simulink model "Case_1"  (R2023b)
settings: Solver=VariableStepAuto  StartTime=0.0  StopTime=1  FixedStep=Ts  RelTol=1e-3  EnableMultiTasking=on
PreLoadFcn:
  | %% Parameters for BLDC Speed Control Example
  | 
  | % This example shows how to control the rotor speed in a BLDC based
  | % electrical drive. An ideal torque source provides the load. The Control
  | % subsystem uses a PI-based cascade control structure with an outer speed
  | % control loop and an inner dc-link voltage control loop. The dc-link
  | % voltage is adjusted through a DC-DC buck converter. The BLDC is fed by
  | % a controlled three-phase inverter. The gate signals for the inverter
  | % are obtained from hall signals. The simulation uses speed steps. The
  | % Scopes subsystem contains scopes that allow you to see the simulation
  | % results.
  | 
  | % Copyright 2017 The MathWorks, Inc.
  | 
  | %% Machine Parameters
  | p    = 4;        % Number of pole pairs
  | Rs   = 0.1;      % Stator resistance per phase           [Ohm]
  | Ls   = 1e-4;     % Stator self-inductance per phase, Ls  [H]
  | Ms   = 1e-5;     % Stator mutual inductance, Ms          [H]
  | psim = 0.0175;   % Maximum permanent magnet flux linkage [Wb]
  | Jm   = 0.0005;   % Rotor inertia                         [Kg*m^2]
  | 
  | %% Control Parameters
  | Ts  = 5e-6;  % Fundamental sample time            [s]
  | Tsc = 1e-4;  % Sample time for inner control loop [s]
  | Vdc = 48;    % Maximum DC link voltage            [V]
  | Kpw = 0.1;   % Proportional gain speed controller
  | Kiw = 15;    % Integrator gain speed controller
  | Kpv = 0.1;   % Proportional gain voltage controller
  | Kiv = 0.5;   % Integrator gain voltage controller
libraries: nesl_utility x16, fl_lib x13, ee_lib x6, slctrl_autotuning x2, eeDiscretePi x2, eeGeneralControl x1, eePwmGenerator x1, spsTriangleGeneratorLib x1
CloseFcn:
  | try,close(h1_pe_bldc_speed_control),end
  | clear h1_pe_bldc_speed_control
  | 
  | clear simlog_pe_bldc_speed_control
  | clear logsout_pe_bldc_speed_control
Description:
  | BLDC Speed Control
settings Model: Creator=The MathWorks, Inc.  LastModifiedBy=HP
settings SolverCC: AllowMultiTaskInputOutput=on  AlgebraicLoopSolver=TrustRegion  AutoInsertRateTranBlk=on  MinimalZcImpactIntegration=on  MaxZcPerStep=1
settings DataIOCC: MaxDataPoints=210000  SaveOutput=off  SignalLogging=off  DSMLogging=off  SaveTime=off  SignalLoggingName=logsout_pe_bldc_speed_control
settings OptimizationCC: ReuseModelBlockBuffer=off  LifeSpan=inf
settings DebuggingCC: UnderspecifiedInitializationDetection=Classic  MergeDetectMultiDrivingBlocksExec=none  UnconnectedInputMsg=warning  UnconnectedOutputMsg=warning  UnconnectedLineMsg=warning  PregeneratedLibrarySubsystemCodeDiagnostic=none  SFUnexpectedBacktrackingDiag=warning  SFNoUnconditionalDefaultTransitionDiag=warning  SFExecutionAtInitializationDiag=none  ArithmeticOperatorsInVariantConditions=warning
settings ModelReferenceCC: EnableRefExpFcnMdlSchedulingChecks=on
settings SFSimCC: SimUseLocalCustomCode=off  CustomCodeUndefinedFunction=UseInterfaceOnly
settings RTWCC: RTWUseLocalCustomCode=off  CheckMdlBeforeBuild=Warning  DLArmComputeVersion=19.05
settings CodeAppCC: StateflowObjectComments=on
settings ConfigComp: CovMetricSettings=dw  CovSaveCumulativeToWorkspaceVar=on  CovSaveSingleToWorkspaceVar=on  CovExternalEMLEnable=off
settings SimscapeCC: SimscapeNormalizeSystem=off  SimscapeLogSimulationStatistics=on  SimscapeLogName=simlog_pe_bldc_speed_control  SimscapeLogDataHistory=210000

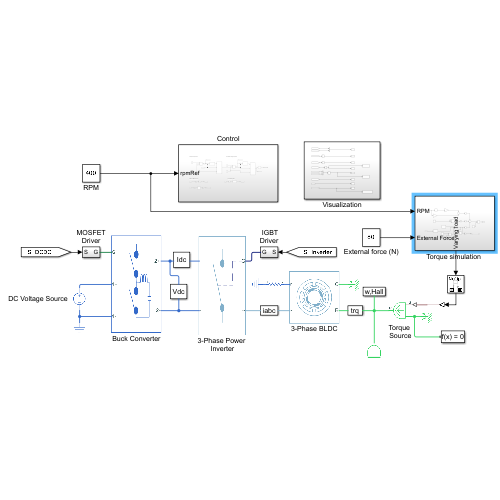
[thumbnail: Simulink's stored preview of the top-level diagram]
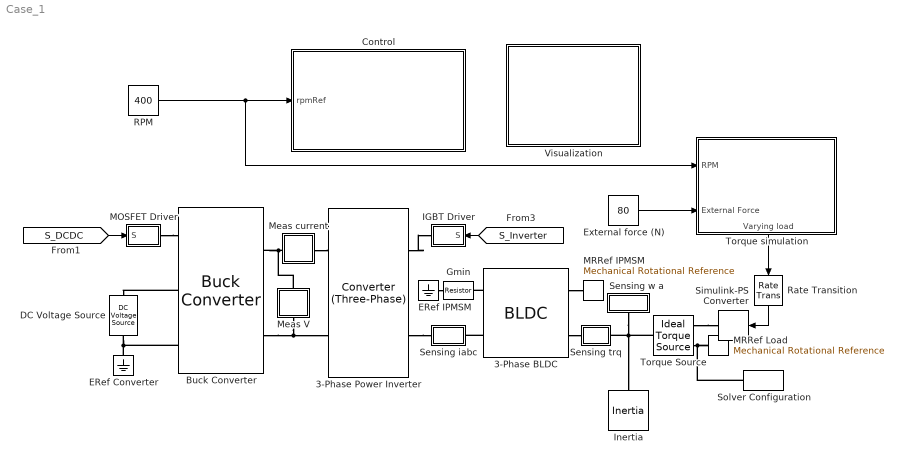
== system Case_1 ==
  " DC Voltage Source" : fl_lib/Electrical/Electrical Sources/DC Voltage Source  v0=Vdc V
  " IGBT Driver" : Subsystem
  3-Phase BLDC : ee_lib/Electromechanical/Permanent Magnet/BLDC  port_option=ee.enum.threePhasePort.composite  rotor_param=1  pm_flux_linkage=psim Wb  theta_constant=pi / (2*p) rad  emf_max=9.6 V  w_meas=600 rpm  DphiDtheta_tab=[0, -.1528, -.1528, .1528, .1528, 0] Wb/rad  back_emf_tab=[0, -9.6, -9.6, 9.6, 9.6, 0] V  rotor_angle_tab=[0, 7.5, 22.5, 37.5, 52.5, 60] deg  nPolePairs=p  axes_param=1  winding_type=ee.enum.statorconnection.wye  stator_param=2  machine_param=ee.enum.dqparameterization.constant  Ld=0.00022 H  Lq=0.00022 H  idVec=[-200, 0, 200] A  iqVec=[-200, 0, 200] A  LdMatrix=0.00022 * ones(3, 3) H  LqMatrix=0.00022 * ones(3, 3) H  L0=0.00016 H  Ls=Ls H  Lm=0 H  Ms=Ms H  Rs=Rs Ohm  zero_sequence=ee.enum.park.zerosequence.include  loss_param=ee.enum.ironloss.none  losses_oc=[0, 0, 0] W  losses_sc=[0, 0, 0] W  f_losses=60 Hz  Isc_losses=95 A  J=0.01 kg*m^2  lam=0 N*m/(rad/s)  i_d_specify=off  i_d_priority=None  i_d=0 A  i_d_nominal_specify=off  i_d_nominal_unit=A  i_d_nominal_value=1  i_q_specify=off  i_q_priority=None  i_q=0 A  i_q_nominal_specify=off  i_q_nominal_unit=A  i_q_nominal_value=1  torque_specify=off  torque_priority=None  torque=0 N*m  torque_nominal_specify=off  torque_nominal_unit=N*m  torque_nominal_value=1  angular_velocity_specify=off  angular_velocity_priority=High  angular_velocity=0 rpm  angular_velocity_nominal_specify=off  angular_velocity_nominal_unit=rpm  angular_velocity_nominal_value=1  angular_position_specify=off  angular_position_priority=High  angular_position=0 deg  angular_position_nominal_specify=off  angular_position_nominal_unit=deg  angular_position_nominal_value=1  alpha=3.93e-3 1/K  alpha_flux=-0.001 1/K  Tmeas=298.15 K  stator_thermal_mass=100 J/K  rotor_thermal_mass=200 J/K  Rm_percent_rotor=90  Rd_percent_rotor=30  temperatureA_specify=off  temperatureA_priority=High  temperatureA=25 degC  temperatureA_nominal_specify=off  temperatureA_nominal_unit=degC  temperatureA_nominal_value=1  temperatureB_specify=off  temperatureB_priority=High  temperatureB=25 degC  temperatureB_nominal_specify=off  temperatureB_nominal_unit=degC  temperatureB_nominal_value=1  temperatureC_specify=off  temperatureC_priority=High  temperatureC=25 degC  temperatureC_nominal_specify=off  temperatureC_nominal_unit=degC  temperatureC_nominal_value=1  temperatureR_specify=off  temperatureR_priority=High  temperatureR=25 degC  temperatureR_nominal_specify=off  temperatureR_nominal_unit=degC  temperatureR_nominal_value=1
      settings: InternalSimscapePortConfiguration="{\"Bottom\":[],\"Left\":[{\"id\":\"N\",\"label\":\"~\",\"type\":\"foundation.electrical.three_phase\"},{\"id\":\"n\",\"label\":\"n\",\"type\":\"foundation.electrical.electrical\"}],\"Right\":[{\"id\":\"R\",\"label\":\"R\",\"type\":\"foundation.mechanical.rotational.rotational\"},{\"id\":\"C\",\"label\":\"C\",\"type\":\"foundation.mechanical.rotational.rotational\"}],\"Top\":[]}"
  3-Phase Power Inverter : ee_lib/Semiconductors & Converters/Converters/Converter (Three-Phase)  port_option=ee.enum.threePhasePort.composite  device_type=3  K=0  Vf=0.8 V  Ron=0.001 Ohm  Rds=0.001 Ohm  Goff=1e-5 1/Ohm  Vgt=1 V  Vgt_off=-1 V  Ih=1 A  Vth=0.5 V  diode_param=2  diode_Vf=0.8 V  diode_Ron=0.001 Ohm  diode_Goff=1e-5 1/Ohm  diode_C=50 nF  diode_iRM=-235 A  diode_iF=300 A  diode_idot=-50 A/us  diode_trr_param=1  diode_trr_factor=3  diode_trr=15 us  diode_Qrr=1.5e+3 s*uA  snubber_type=0  Cs=1e-7 F  Rs=0.1 Ohm
  Buck Converter : ee_lib/Semiconductors & Converters/Converters/Buck Converter  port_option=ee.enum.controlport.ps  device_type=4  Vf=0.8 V  Ron=0.001 Ohm  Rds=0.001 Ohm  Goff=1e-5 1/Ohm  Vgt=1 V  Vgt_off=-1 V  Ih=1 A  Vth=0.5 V  K=0  diode_param=2  diode_Vf=0.8 V  diode_Ron=0.001 Ohm  diode_Goff=1e-5 1/Ohm  diode_C=50 nF  diode_iRM=-235 A  diode_iF=300 A  diode_idot=-50 A/us  diode_trr_param=1  diode_trr_factor=3  diode_trr=15 us  diode_Qrr=1500 s*uA  Lf=220 uH  Rl=0 Ohm  Cf=10 uF  Rf=.25 Ohm  snubber_type=1  Cs=1e-7 F  Rs=0.1 Ohm  iL_specify=off  iL_priority=High  iL=0 A  iL_nominal_specify=off  iL_nominal_unit=A  iL_nominal_value=1  vc_specify=off  vc_priority=High  vc=0 V  vc_nominal_specify=off  vc_nominal_unit=V  vc_nominal_value=1
      settings: InternalSimscapePortConfiguration="{\"Bottom\":[],\"Left\":[{\"id\":\"G\",\"label\":\"G\",\"type\":\"foundation.electrical.four_phase\"},{\"id\":\"p1\",\"label\":\"1+\",\"type\":\"foundation.electrical.electrical\"},{\"id\":\"n1\",\"label\":\"1-\",\"type\":\"foundation.electrical.electrical\"}],\"Right\":[{\"id\":\"p2\",\"label\":\"2+\",\"type\":\"foundation.electrical.electrical\"},{\"id\":\"n2\",\"label\":\"2-\",\"type\":\"foundation.electrical.electrical\"}],\"Top\":[]}"
  Control : Subsystem
  ERef Converter : fl_lib/Electrical/Electrical Elements/Electrical Reference
  ERef IPMSM : fl_lib/Electrical/Electrical Elements/Electrical Reference
  External force (N) : Constant  Value=80
  Gmin : fl_lib/Electrical/Electrical Elements/Resistor  R=1e9 Ohm  i_specify=off  i_priority=High  i=0 A  i_nominal_specify=off  i_nominal_unit=A  i_nominal_value=1  v_specify=off  v_priority=High  v=0 V  v_nominal_specify=off  v_nominal_unit=V  v_nominal_value=1
  Inertia : fl_lib/Mechanical/Rotational Elements/Inertia  inertia=Jm kg*m^2  num_ports=foundation.enum.numPorts2.one  w_specify=on  w_priority=High  w=0 rpm  w_nominal_specify=off  w_nominal_unit=rad/s  w_nominal_value=1  t_specify=off  t_priority=High  t=0 N*m  t_nominal_specify=off  t_nominal_unit=N*m  t_nominal_value=1
  "MOSFET Driver " : Subsystem
  MRRef IPMSM : fl_lib/Mechanical/Rotational Elements/Mechanical Rotational Reference
  MRRef Load : fl_lib/Mechanical/Rotational Elements/Mechanical Rotational Reference
  Meas V : Subsystem
      mask Display: disp('Vdc')
  Meas current : Subsystem
      settings: PortSchema="{\"entries\":[{\"content\":{\"sides\":[{\"content\":{},\"type\":\"ConnectorPlacement.EquallySpacedRectSide\",\"uuid\":\"82ca6d8b-4f1d-482c-9132-345f1111dd8f\"},{\"content\":{\"side\":\"RIGHT\"},\"type\":\"ConnectorPlacement.EquallySpacedRectSide\",\"uuid\":\"46eb7c2e-5f99-46a8-b5a6-ad4c053dfe5d\"},{\"content\":{\"connectorIds\":[\"LConn1\"],\"side\":\"TOP\"},\"type\":\"ConnectorPlacement.EquallySpacedRectSide\",\"uuid\":\"5837dc94-a870-4fd0-9d92-a25376552da6\"},{\"content\":{\"connectorIds\":[\"RConn1\"],\"side\":\"BOTTOM\"},\"type\":\"ConnectorPlacement.EquallySpacedRectSide\",\"uuid\":\"ef4e5c2a-3af4-4835-9bd1-a57a6b683b63\"}]},\"type\":\"ConnectorPlacement.EquallySpacedConnector\",\"uuid\":\"b19ad980-4c6f-4f24-94cb-fca13afdc426\"}],\"packageUris\":[\"http://schema.mathworks.com/mf0/Connector/R2020b\"],\"version\":\"1.0\"}"
      mask Display: disp('Idc')
  RPM : Constant  Value=400
  Rate Transition : RateTransition  OutPortSampleTimeOpt=Inherit
  Sensing trq : Subsystem
      mask Display: disp('trq')
  Sensing w a : Subsystem
      mask Display: disp('w,Hall')
  Sensing iabc : Subsystem
      mask Display: disp('iabc')
  Simulink-PS Converter : nesl_utility/Simulink-PS Converter  PhysicalDomain=network_engine_domain  SubClassName=ps_input  LeftPortType=input  RightPortType=output  PseudoPeriodic=off  Frequencies=[]  NoiseDistribution=none  NoiseParameters=[]  Unit=N*m  AffineConversion=on  FilteringAndDerivatives=zero  SimscapeFilterOrder=1  InputFilterTimeConstant=0.001  UdotUserProvided=1
  Solver Configuration : nesl_utility/Solver Configuration  PhysicalDomain=network_engine_domain  SubClassName=solver  LeftPortType=input  RightPortType=generic  Tones=[]  Harmonics=[]  SimulateNoise=off  Profile=off  UseLocalSampling=off  EnableSwitchedLinearOptims=on  FrequencyDomain=off  UseCCode=off  RelTol=0.001  AbsTol=1e-06  MinStep=1e-09  ToWorkspace=off  RevertToSquareIcSolve=off  NumHomotopyIterations=100  PhasorMode=off  PhasorModeNumHarmonics=1  ConsistencySolver=NEWTON_FTOL  IndexReductionMethod=DerivativeReplacement  DoDC=off  ResidualTolerance=1e-9  ConsistencyTolSource=GLOBAL  ConsistencyAbsTol=0.001  ConsistencyRelTol=0.001  ConsistencyTolFactor=0.001  UseLocalSolver=on  LocalSolverChoice=NE_BACKWARD_EULER_ADVANCER  ResolveIndetEquations=on  FunctionEvalNumThread=1  LocalSolverSampleTime=Ts  DoFixedCost=on  MaxNonlinIter=4  MaxModeIter=2  ComputeImpulses=off  ImpulseIterations=2  LinearAlgebra=Sparse  LinearAlgebraNumThread=0  EquationFormulation=NE_TIME_EF  DelaysMemoryBudget=1024  AutomaticFiltering=on  FilteringTimeConstant=0.001  PartitionStorageMethod=AS_NEEDED  PartitionMemoryBudget=1024  PartitionMethod=FAST  MultibodyUseLocalSolver=off  MultibodyLocalSolverChoice=ODE1  MultibodyLocalSolverSampleTime=0.001
  Torque Source : fl_lib/Mechanical/Mechanical Sources/Ideal Torque Source
  "Torque simulation " : Subsystem
      settings: PortSchema="{\"entries\":[{\"content\":{\"sides\":[{\"content\":{\"connectorIds\":[\"In1\",\"In2\"]},\"type\":\"ConnectorPlacement.EquallySpacedRectSide\",\"uuid\":\"4de94c05-994b-4a6b-aa57-8a8325026801\"},{\"content\":{\"side\":\"RIGHT\"},\"type\":\"ConnectorPlacement.EquallySpacedRectSide\",\"uuid\":\"9aab4c8e-5a08-4361-b962-7ff1ea4c45cd\"},{\"content\":{\"side\":\"TOP\"},\"type\":\"ConnectorPlacement.EquallySpacedRectSide\",\"uuid\":\"3907e8e7-ade8-4b6d-b9e3-a2c225338252\"},{\"content\":{\"connectorIds\":[\"Out1\"],\"side\":\"BOTTOM\"},\"type\":\"ConnectorPlacement.EquallySpacedRectSide\",\"uuid\":\"9adc3eea-f106-4f90-8d03-70cb44881ebc\"}]},\"type\":\"ConnectorPlacement.EquallySpacedConnector\",\"uuid\":\"d6098bb0-da6b-4857-a7db-fd24669e7041\"}],\"packageUris\":[\"http://schema.mathworks.com/mf0/Connector/R2020b\"],\"version\":\"1.0\"}"
  Visualization : Subsystem
  wires:
  [S_DCDC] -> "MOSFET Driver "/1(S)
  [S_Inverter] -> " IGBT Driver"/1(S)
  "Torque simulation "/1(Varying load) -> Rate Transition/1
  External force (N)/1 -> "Torque simulation "/2(External Force)
  RPM/1 -> "Torque simulation "/1(RPM), Control/1(rpmRef)
  Rate Transition/1 -> Simulink-PS Converter/1
  connections:
  Torque Source/LConn1 -- Sensing w a/LConn1 -- Sensing trq/RConn1 -- Inertia/LConn1
  ERef IPMSM/LConn1 -- Gmin/LConn1
  3-Phase BLDC/LConn2 -- Gmin/RConn1
  Torque Source/RConn1 -- Simulink-PS Converter/RConn1
  Torque Source/RConn2 -- Solver Configuration/RConn1 -- MRRef Load/LConn1
  3-Phase BLDC/LConn1 -- Sensing iabc/RConn1
  3-Phase BLDC/RConn2 -- MRRef IPMSM/LConn1
  3-Phase BLDC/RConn1 -- Sensing trq/LConn1
  Buck Converter/LConn2 -- " DC Voltage Source"/LConn1
  ERef Converter/LConn1 -- " DC Voltage Source"/RConn1 -- Buck Converter/LConn3
  "MOSFET Driver "/RConn1 -- Buck Converter/LConn1
  Buck Converter/RConn2 -- Meas V/RConn1 -- 3-Phase Power Inverter/RConn2
  Meas V/LConn1 -- Meas current/LConn1 -- Buck Converter/RConn1
  3-Phase Power Inverter/LConn1 -- " IGBT Driver"/RConn1
  3-Phase Power Inverter/LConn2 -- Sensing iabc/LConn1
  Meas current/RConn1 -- 3-Phase Power Inverter/RConn1

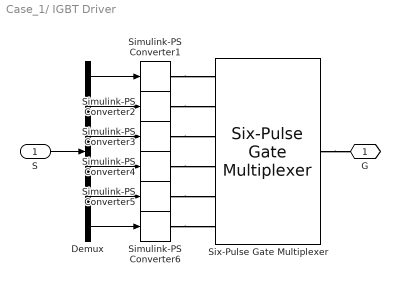
== system Case_1/ IGBT Driver ==
  S : Inport
  Demux : Demux  Outputs=6
  Simulink-PS Converter{1..6} (6 alike) : nesl_utility/Simulink-PS Converter  PhysicalDomain=network_engine_domain  SubClassName=ps_input  LeftPortType=input  RightPortType=output  PseudoPeriodic=off  Frequencies=[]  NoiseDistribution=none  NoiseParameters=[]  Unit=1  AffineConversion=off  FilteringAndDerivatives=zero  SimscapeFilterOrder=1  InputFilterTimeConstant=0.001  UdotUserProvided=1
  Six-Pulse Gate Multiplexer : ee_lib/Semiconductors & Converters/Converters/Six-Pulse Gate Multiplexer  port_option=ee.enum.controlport.ps
  G : PMIOPort  Side=Right
  wires:
  Demux/1 -> Simulink-PS Converter1/1
  S/1 -> Demux/1
  Demux/4 -> Simulink-PS Converter4/1
  Demux/2 -> Simulink-PS Converter2/1
  Demux/3 -> Simulink-PS Converter3/1
  Demux/5 -> Simulink-PS Converter5/1
  Demux/6 -> Simulink-PS Converter6/1
  connections:
  Six-Pulse Gate Multiplexer/RConn1 -- G/RConn1
  Simulink-PS Converter1/RConn1 -- Six-Pulse Gate Multiplexer/LConn1
  Simulink-PS Converter3/RConn1 -- Six-Pulse Gate Multiplexer/LConn3
  Simulink-PS Converter5/RConn1 -- Six-Pulse Gate Multiplexer/LConn5
  Simulink-PS Converter6/RConn1 -- Six-Pulse Gate Multiplexer/LConn6
  Simulink-PS Converter4/RConn1 -- Six-Pulse Gate Multiplexer/LConn4
  Simulink-PS Converter2/RConn1 -- Six-Pulse Gate Multiplexer/LConn2

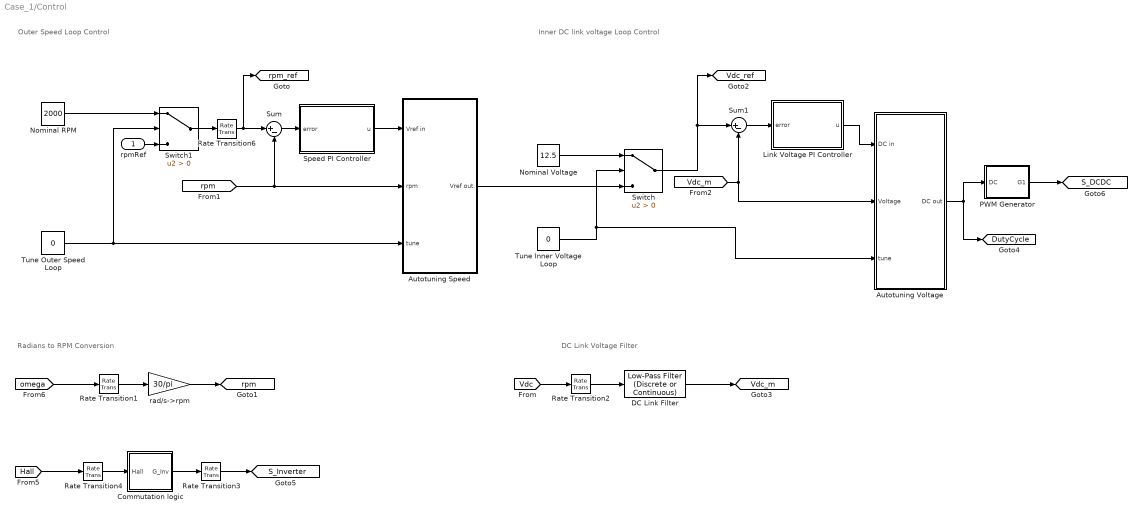
== system Case_1/Control ==
  note: Inner DC link voltage Loop Control
  note: Outer Speed Loop Control
  note: DC Link Voltage Filter
  note: Radians to RPM Conversion
  rpmRef : Inport
  Autotuning Speed : Subsystem
  Autotuning Voltage : Subsystem
  Commutation logic : Subsystem
  DC Link Filter : eeGeneralControl/Low-Pass Filter (Discrete or Continuous)  K=1  T=0.01  B=inf  A=-inf  init_option=Inherited from block input  x0=0  Ts=Tsc
  Link Voltage PI Controller : Subsystem
  Nominal RPM : Constant  Value=2000
  Nominal Voltage : Constant  Value=12.5
  PWM Generator : Subsystem
  Rate Transition1 : RateTransition
  Rate Transition2 : RateTransition
  Rate Transition3 : RateTransition  OutPortSampleTime=Ts
  Rate Transition4 : RateTransition  OutPortSampleTime=Tsc
  Rate Transition6 : RateTransition
  Speed PI Controller : Subsystem
  Sum : Sum  Inputs=|+-
  Sum1 : Sum  Inputs=|+-
  Switch : Switch  Criteria=u2 > Threshold  SaturateOnIntegerOverflow=off  InputSameDT=off
  Switch1 : Switch  Criteria=u2 > Threshold  SaturateOnIntegerOverflow=off  InputSameDT=off
  Tune Inner Voltage Loop : Constant  Value=0
  Tune Outer Speed Loop : Constant  Value=0
  rad/s->rpm : Gain  Gain=30/pi
  tag scope: DutyCycle=global, S_DCDC=global, S_Inverter=global, Vdc_m=global, Vdc_ref=global, rpm=global, rpm_ref=global
  wires:
  [omega] -> Rate Transition1/1
  [Hall] -> Rate Transition4/1
  rpmRef/1 -> Switch1/3
  Rate Transition6/1 -> [rpm_ref], Sum/1
  Rate Transition1/1 -> rad/s->rpm/1
  rad/s->rpm/1 -> [rpm]
  Rate Transition3/1 -> [S_Inverter]
  Rate Transition4/1 -> Commutation logic/1(Hall)
  Commutation logic/1(G_Inv) -> Rate Transition3/1
  PWM Generator/1(G1) -> [S_DCDC]
  [Vdc] -> Rate Transition2/1
  Autotuning Voltage/1(DC out) -> PWM Generator/1(DC), [DutyCycle]
  Rate Transition2/1 -> DC Link Filter/1
  DC Link Filter/1 -> [Vdc_m]
  Nominal Voltage/1 -> Switch/1
  Switch1/1 -> Rate Transition6/1
  Nominal RPM/1 -> Switch1/1
  Tune Inner Voltage Loop/1 -> Autotuning Voltage/3(tune), Switch/2
  Autotuning Speed/1(Vref out) -> Switch/3
  Tune Outer Speed Loop/1 -> Switch1/2, Autotuning Speed/3(tune)
  [rpm] -> Sum/2, Autotuning Speed/2(rpm)
  [Vdc_m] -> Sum1/2, Autotuning Voltage/2(Voltage)
  Sum/1 -> Speed PI Controller/1(error)
  Speed PI Controller/1(u) -> Autotuning Speed/1(Vref in)
  Link Voltage PI Controller/1(u) -> Autotuning Voltage/1(DC in)
  Sum1/1 -> Link Voltage PI Controller/1(error)
  Switch/1 -> Sum1/1, [Vdc_ref]

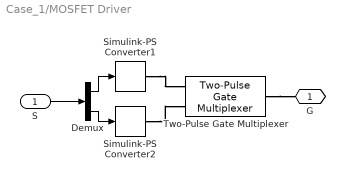
== system Case_1/MOSFET Driver  ==
  S : Inport
  Demux : Demux  Outputs=2
  Simulink-PS Converter1 : nesl_utility/Simulink-PS Converter  PhysicalDomain=network_engine_domain  SubClassName=ps_input  LeftPortType=input  RightPortType=output  PseudoPeriodic=off  Frequencies=[]  NoiseDistribution=none  NoiseParameters=[]  Unit=V  AffineConversion=off  FilteringAndDerivatives=zero  SimscapeFilterOrder=1  InputFilterTimeConstant=0.001  UdotUserProvided=1
  Simulink-PS Converter2 : nesl_utility/Simulink-PS Converter  PhysicalDomain=network_engine_domain  SubClassName=ps_input  LeftPortType=input  RightPortType=output  PseudoPeriodic=off  Frequencies=[]  NoiseDistribution=none  NoiseParameters=[]  Unit=V  AffineConversion=off  FilteringAndDerivatives=zero  SimscapeFilterOrder=1  InputFilterTimeConstant=0.001  UdotUserProvided=1
  Two-Pulse Gate Multiplexer : ee_lib/Semiconductors & Converters/Converters/Two-Pulse Gate Multiplexer  port_option=ee.enum.controlport.ps
      settings: InternalSimscapePortConfiguration="{\"Bottom\":[],\"Left\":[{\"id\":\"G1_ps\",\"label\":\"G1\",\"type\":\"input\"},{\"id\":\"G2_ps\",\"label\":\"G2\",\"type\":\"input\"}],\"Right\":[{\"id\":\"p\",\"label\":\"G\",\"type\":\"foundation.electrical.four_phase\"}],\"Top\":[]}"
  G : PMIOPort  Side=Right
  wires:
  Demux/1 -> Simulink-PS Converter1/1
  Demux/2 -> Simulink-PS Converter2/1
  S/1 -> Demux/1
  connections:
  Two-Pulse Gate Multiplexer/RConn1 -- G/RConn1
  Simulink-PS Converter1/RConn1 -- Two-Pulse Gate Multiplexer/LConn1
  Simulink-PS Converter2/RConn1 -- Two-Pulse Gate Multiplexer/LConn2

== system Case_1/Meas V ==
  PS-Simulink Converter2 : nesl_utility/PS-Simulink Converter  PhysicalDomain=network_engine_domain  SubClassName=ps_output  LeftPortType=input  RightPortType=output  PseudoPeriodic=off  Frequencies=[]  VectorFormat=1-D array  Unit=V  AffineConversion=off
  Voltage Sensor : fl_lib/Electrical/Electrical Sensors/Voltage Sensor
  + : PMIOPort  Side=Left
  - : PMIOPort  Port=2  Side=Right
  tag scope: Vdc=global
  wires:
  PS-Simulink Converter2/1 -> [Vdc]
  connections:
  Voltage Sensor/LConn1 -- +/RConn1
  PS-Simulink Converter2/LConn1 -- Voltage Sensor/RConn1
  Voltage Sensor/RConn2 -- -/RConn1

== system Case_1/Meas current ==
  Current Sensor : fl_lib/Electrical/Electrical Sensors/Current Sensor
  PS-Simulink Converter1 : nesl_utility/PS-Simulink Converter  PhysicalDomain=network_engine_domain  SubClassName=ps_output  LeftPortType=input  RightPortType=output  PseudoPeriodic=off  Frequencies=[]  VectorFormat=1-D array  Unit=A  AffineConversion=off
  + : PMIOPort  Side=Left
  - : PMIOPort  Port=2  Side=Right
  tag scope: i=global
  wires:
  PS-Simulink Converter1/1 -> [i]
  connections:
  Current Sensor/LConn1 -- +/RConn1
  Current Sensor/RConn2 -- -/RConn1
  Current Sensor/RConn1 -- PS-Simulink Converter1/LConn1

== system Case_1/Sensing trq ==
  PS-Simulink Converter3 : nesl_utility/PS-Simulink Converter  PhysicalDomain=network_engine_domain  SubClassName=ps_output  LeftPortType=input  RightPortType=output  PseudoPeriodic=off  Frequencies=[]  VectorFormat=1-D array  Unit=N*m  AffineConversion=off
  Torque Sensor : fl_lib/Mechanical/Mechanical Sensors/Ideal Torque Sensor
  R : PMIOPort  Side=Left
  C : PMIOPort  Port=2  Side=Right
  tag scope: TqMeas=global
  wires:
  PS-Simulink Converter3/1 -> [TqMeas]
  connections:
  Torque Sensor/RConn1 -- C/RConn1
  Torque Sensor/RConn2 -- PS-Simulink Converter3/LConn1
  Torque Sensor/LConn1 -- R/RConn1

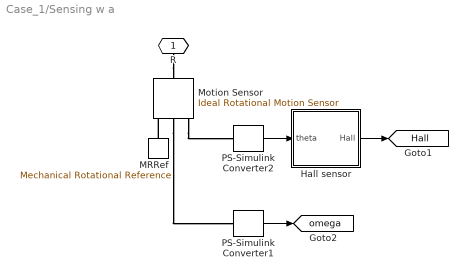
== system Case_1/Sensing w a ==
  Hall sensor : Subsystem
  MRRef : fl_lib/Mechanical/Rotational Elements/Mechanical Rotational Reference
  Motion Sensor : fl_lib/Mechanical/Mechanical Sensors/Ideal Rotational Motion Sensor  reference=foundation.enum.MeasurementReference.difference  acceleration_port=false  velocity_port=true  position_port=true  wrap_angle=simscape.enum.onoff.off  offset=0 deg
  PS-Simulink Converter1 : nesl_utility/PS-Simulink Converter  PhysicalDomain=network_engine_domain  SubClassName=ps_output  LeftPortType=input  RightPortType=output  PseudoPeriodic=off  Frequencies=[]  VectorFormat=1-D array  Unit=rad/s  AffineConversion=off
  PS-Simulink Converter2 : nesl_utility/PS-Simulink Converter  PhysicalDomain=network_engine_domain  SubClassName=ps_output  LeftPortType=input  RightPortType=output  PseudoPeriodic=off  Frequencies=[]  VectorFormat=1-D array  Unit=rad  AffineConversion=off
  R : PMIOPort  Side=Left
  tag scope: Hall=global, omega=global
  wires:
  PS-Simulink Converter1/1 -> [omega]
  PS-Simulink Converter2/1 -> Hall sensor/1(theta)
  Hall sensor/1(Hall) -> [Hall]
  connections:
  R/RConn1 -- Motion Sensor/LConn1
  Motion Sensor/RConn2 -- PS-Simulink Converter1/LConn1
  MRRef/LConn1 -- Motion Sensor/RConn1
  Motion Sensor/RConn3 -- PS-Simulink Converter2/LConn1

== system Case_1/Sensing iabc ==
  Current Sensor : ee_lib/Sensors & Transducers/Current Sensor (Three-Phase)
  PS-Simulink Converter : nesl_utility/PS-Simulink Converter  PhysicalDomain=network_engine_domain  SubClassName=ps_output  LeftPortType=input  RightPortType=output  PseudoPeriodic=off  Frequencies=[]  VectorFormat=1-D array  Unit=A  AffineConversion=off
  1 : PMIOPort  Side=Left
  2 : PMIOPort  Port=2  Side=Right
  tag scope: iabc=global
  wires:
  PS-Simulink Converter/1 -> [iabc]
  connections:
  1/RConn1 -- Current Sensor/LConn1
  2/RConn1 -- Current Sensor/RConn2
  Current Sensor/RConn1 -- PS-Simulink Converter/LConn1

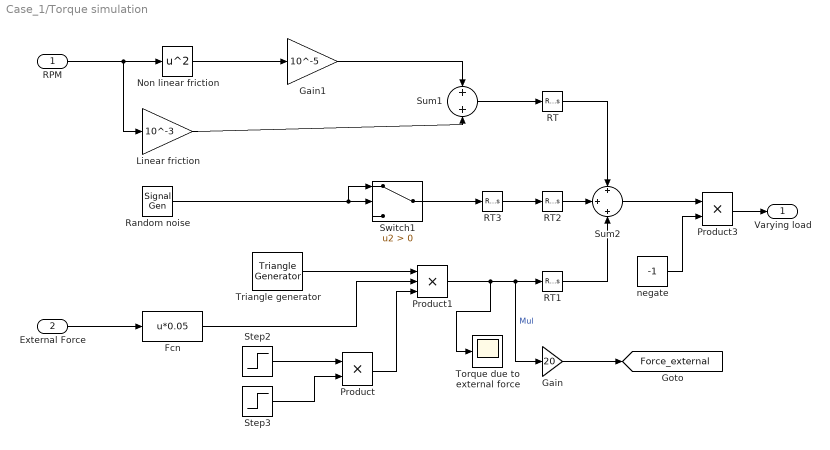
== system Case_1/Torque simulation  ==
  RPM : Inport
  External Force : Inport  Port=2
  Fcn : Fcn  Expr=u*0.05
  Gain : Gain  Gain=20
  Gain1 : Gain  Gain=10^-5
  Linear friction : Gain  Gain=10^-3
  Non linear friction : Math  Operator=square
  Product : Product
  Product1 : Product  Inputs=3
  Product3 : Product
  RT : RateTransition  OutPortSampleTime=1e-03
  RT1 : RateTransition  OutPortSampleTime=1e-03
  RT2 : RateTransition  OutPortSampleTime=1e-03
  RT3 : RateTransition  OutPortSampleTime=0.5e-02
  "Random noise " : SignalGenerator  WaveForm=random  Amplitude=0.5  Frequency=0.5
  Step2 : Step  Time=0.5  SampleTime=0
  Step3 : Step  Time=0.75  Before=1  After=0  SampleTime=0
  Sum1 : Sum  Inputs=+|+
  Sum2 : Sum  Inputs=+|+|+
  Switch1 : Switch  Criteria=u2 > Threshold  SaturateOnIntegerOverflow=off  InputSameDT=off
  Torque due to external force : Scope
  Triangle generator : spsTriangleGeneratorLib/Triangle Generator  Freq=1  Phase=-90  Ts=0
  negate : Constant  Value=-1
  Varying load : Outport
  tag scope: Force_external=global
  wires:
  Gain1/1 -> Sum1/1
  "Random noise "/1 -> Switch1/2, Switch1/1
  RPM/1 -> Linear friction/1, Non linear friction/1
  Product1/1 -> Torque due to external force/1, RT1/1, Gain/1  "Mul"
  Sum2/1 -> Product3/1
  RT1/1 -> Sum2/3
  Sum1/1 -> RT/1
  Non linear friction/1 -> Gain1/1
  External Force/1 -> Fcn/1
  negate/1 -> Product3/2
  Product3/1 -> Varying load/1
  Linear friction/1 -> Sum1/2
  Switch1/1 -> RT3/1
  RT3/1 -> RT2/1
  Product/1 -> Product1/3
  Step3/1 -> Product/2
  Triangle generator/1 -> Product1/1
  Step2/1 -> Product/1
  Fcn/1 -> Product1/2
  RT/1 -> Sum2/1
  Gain/1 -> [Force_external]
  RT2/1 -> Sum2/2

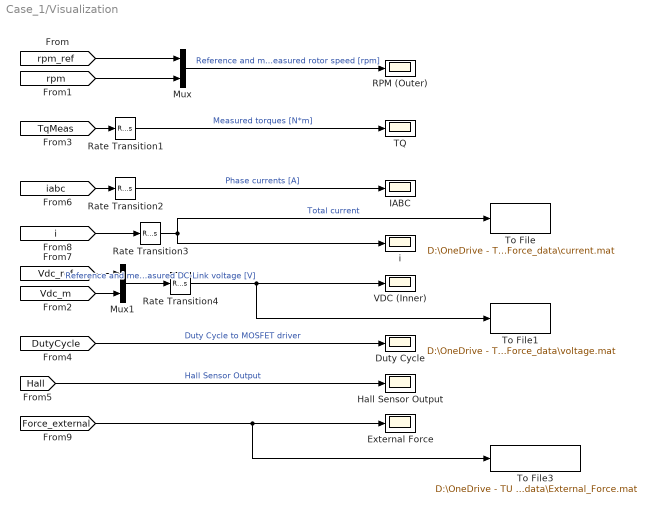
== system Case_1/Visualization ==
  Duty Cycle : Scope
  External Force : Scope
  Hall Sensor Output : Scope
  IABC : Scope
  Mux : Mux  Inputs=2
  Mux1 : Mux  Inputs=2
  RPM (Outer) : Scope
  Rate Transition1 : RateTransition
  Rate Transition2 : RateTransition  OutPortSampleTime=1e-3
  Rate Transition3 : RateTransition  OutPortSampleTime=1e-3
  Rate Transition4 : RateTransition  OutPortSampleTime=1e-3
  TQ : Scope
  To File : ToFile  Filename=D:\OneDrive - TU Eindhoven\5ARIP0_Interdisciplinary Team Project\Data Generation\Current_Volt_Force_data\current.mat  MatrixName=i  SaveFormat=Timeseries
  To File1 : ToFile  Filename=D:\OneDrive - TU Eindhoven\5ARIP0_Interdisciplinary Team Project\Data Generation\Current_Volt_Force_data\voltage.mat  MatrixName=v  SaveFormat=Timeseries
  To File3 : ToFile  Filename=D:\OneDrive - TU Eindhoven\5ARIP0_Interdisciplinary Team Project\Data Generation\Current_Volt_Force_data\External_Force.mat  MatrixName=force  SaveFormat=Timeseries
  VDC (Inner) : Scope
  i : Scope
  wires:
  [rpm] -> Mux/2
  [Vdc_ref] -> Mux1/1
  Rate Transition2/1 -> IABC/1  "Phase currents [A]"
  [rpm_ref] -> Mux/1
  [iabc] -> Rate Transition2/1
  [TqMeas] -> Rate Transition1/1
  Rate Transition1/1 -> TQ/1  "Measured torques [N*m]"
  Mux/1 -> RPM (Outer)/1  "Reference and measured rotor speed [rpm]"
  [Vdc_m] -> Mux1/2
  [DutyCycle] -> Duty Cycle/1  "Duty Cycle to MOSFET driver"
  [Hall] -> Hall Sensor Output/1  "Hall Sensor Output"
  [i] -> Rate Transition3/1
  Rate Transition3/1 -> To File/1, i/1  "Total current"
  Mux1/1 -> Rate Transition4/1  "Reference and measured DC-Link voltage [V]"
  Rate Transition4/1 -> To File1/1, VDC (Inner)/1
  [Force_external] -> To File3/1, External Force/1

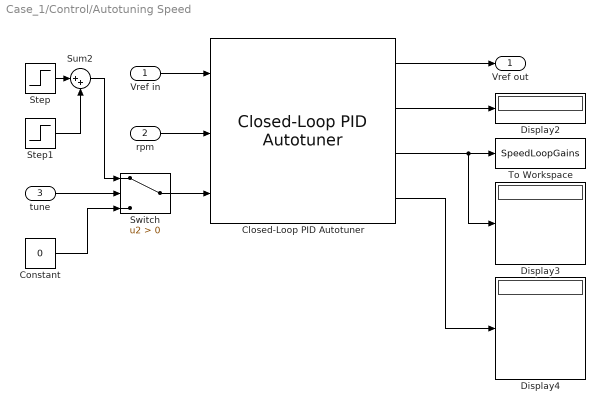
== system Case_1/Control/Autotuning Speed ==
  Vref in : Inport
  rpm : Inport  Port=2
  tune : Inport  Port=3
  Closed-Loop PID Autotuner : slctrl_autotuning/Closed-Loop PID Autotuner  PIDType=PID  PIDForm=Parallel  TimeDomain=discrete-time  DiscreteTs=Tsc  TuningTs=0.2  UseTuningTs=off  IntegratorFormula=Forward Euler  FilterFormula=Forward Euler  ContinuousTs=0.02  Bandwidth=100  UseExternalWC=off  TargetPM=60  UseExternalPM=off  UseExternalAchievedPM=off  ExperimentMode=Superposition  PlantType=Stable  PlantSign=Positive  AmpSine=1  UseExternalAmpSine=off  UseExternalFRD=on  UseExternalU0=off  UseCompanion=off  NotDeployTuningModule=off  UsePLCCoder=off  OutputMode=control action + perturbation  BlockDataType=double  UseConnectedPID=on  blockpath=[]  tunedP=0  tunedI=0  tunedD=0  tunedN=100  tunedPM=0  EstimationWindowSize=3  UseExternalTuningParams=off  SingleMultiRateVariant=SingleSamplingRate  NumEstimationPeriods=4  NumSettlingPeriods=2  NumOfPRBSPeriod=1  PRBSSignalOrder=12  ExperimentModeVariant=VariantSuperimposed  OutputChoice=VariantCandD
  Constant : Constant  Value=0
  Display2 : Display
  Display3 : Display
  Display4 : Display
  Step : Step  SampleTime=0
  Step1 : Step  Time=1.9  After=-1  SampleTime=0
  Sum2 : Sum  Inputs=|++
  Switch : Switch  Criteria=u2 > Threshold  SaturateOnIntegerOverflow=off  InputSameDT=off
  To Workspace : ToWorkspace  VariableName=SpeedLoopGains  SampleTime=-1
      settings: MaxDataPoints=1
  Vref out : Outport  VectorParamsAs1DForOutWhenUnconnected=off
  wires:
  Closed-Loop PID Autotuner/3 -> To Workspace/1, Display3/1
  Closed-Loop PID Autotuner/4 -> Display4/1
  rpm/1 -> Closed-Loop PID Autotuner/2
  Closed-Loop PID Autotuner/1 -> Vref out/1
  Vref in/1 -> Closed-Loop PID Autotuner/1
  Closed-Loop PID Autotuner/2 -> Display2/1
  Step1/1 -> Sum2/2
  Step/1 -> Sum2/1
  Switch/1 -> Closed-Loop PID Autotuner/3
  Constant/1 -> Switch/3
  tune/1 -> Switch/2
  Sum2/1 -> Switch/1

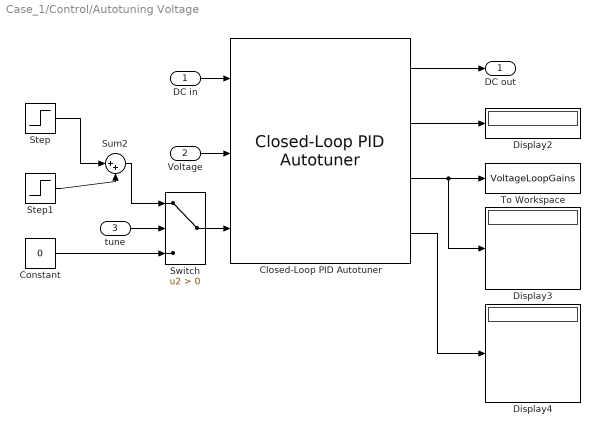
== system Case_1/Control/Autotuning Voltage ==
  DC in : Inport
  Voltage : Inport  Port=2
  tune : Inport  Port=3
  Closed-Loop PID Autotuner : slctrl_autotuning/Closed-Loop PID Autotuner  PIDType=PI  PIDForm=Parallel  TimeDomain=discrete-time  DiscreteTs=Tsc  TuningTs=0.2  UseTuningTs=off  IntegratorFormula=Forward Euler  FilterFormula=Forward Euler  ContinuousTs=0.02  Bandwidth=400  UseExternalWC=off  TargetPM=60  UseExternalPM=off  UseExternalAchievedPM=off  ExperimentMode=Superposition  PlantType=Stable  PlantSign=Positive  AmpSine=0.1  UseExternalAmpSine=off  UseExternalFRD=on  UseExternalU0=off  UseCompanion=off  NotDeployTuningModule=off  UsePLCCoder=off  OutputMode=control action + perturbation  BlockDataType=double  UseConnectedPID=on  blockpath=[]  tunedP=0  tunedI=0  tunedD=0  tunedN=100  tunedPM=0  EstimationWindowSize=3  UseExternalTuningParams=off  SingleMultiRateVariant=SingleSamplingRate  NumEstimationPeriods=4  NumSettlingPeriods=2  NumOfPRBSPeriod=1  PRBSSignalOrder=12  ExperimentModeVariant=VariantSuperimposed  OutputChoice=VariantCandD
  Constant : Constant  Value=0
  Display2 : Display
  Display3 : Display
  Display4 : Display
  Step : Step  SampleTime=0
  Step1 : Step  Time=1.8  After=-1  SampleTime=0
  Sum2 : Sum  Inputs=|++
  Switch : Switch  Criteria=u2 > Threshold  SaturateOnIntegerOverflow=off  InputSameDT=off
  To Workspace : ToWorkspace  VariableName=VoltageLoopGains  SampleTime=-1
      settings: MaxDataPoints=1
  DC out : Outport  VectorParamsAs1DForOutWhenUnconnected=off
  wires:
  Closed-Loop PID Autotuner/3 -> To Workspace/1, Display3/1
  Closed-Loop PID Autotuner/4 -> Display4/1
  Voltage/1 -> Closed-Loop PID Autotuner/2
  DC in/1 -> Closed-Loop PID Autotuner/1
  Step1/1 -> Sum2/2
  Step/1 -> Sum2/1
  Switch/1 -> Closed-Loop PID Autotuner/3
  tune/1 -> Switch/2
  Constant/1 -> Switch/3
  Sum2/1 -> Switch/1
  Closed-Loop PID Autotuner/1 -> DC out/1
  Closed-Loop PID Autotuner/2 -> Display2/1

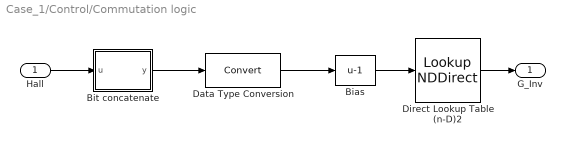
== system Case_1/Control/Commutation logic ==
  Hall : Inport
  Bias : Bias  Bias=-1  SaturateOnIntegerOverflow=off
  Bit concatenate : Subsystem
  Data Type Conversion : DataTypeConversion  SaturateOnIntegerOverflow=off  RndMeth=Floor
  Direct Lookup Table (n-D)2 : LookupNDDirect  InputsSelectThisObjectFromTable=Vector  Table=[0 0 0 1 1 0;0 1 1 0 0 0;0 1 0 0 0 1;1 0 0 0 1 0;1 0 1 0 0 0;0 0 0 1 0 1]
  G_Inv : Outport  VectorParamsAs1DForOutWhenUnconnected=off
  wires:
  Hall/1 -> Bit concatenate/1(u)
  Bit concatenate/1(y) -> Data Type Conversion/1
  Direct Lookup Table (n-D)2/1 -> G_Inv/1
  Data Type Conversion/1 -> Bias/1
  Bias/1 -> Direct Lookup Table (n-D)2/1

== system Case_1/Control/Link Voltage PI Controller ==
  error : Inport
  Constant1 : Constant  Value=0  SampleTime=Tsc
  Voltage controller : eeDiscretePi/Discrete PI Controller with Integral Anti-Windup  Kp=Kpv  Ki=Kiv  x0=0  B=1  A=0  Ts=Tsc
  u : Outport  VectorParamsAs1DForOutWhenUnconnected=off
  wires:
  Constant1/1 -> Voltage controller/2
  error/1 -> Voltage controller/1
  Voltage controller/1 -> u/1

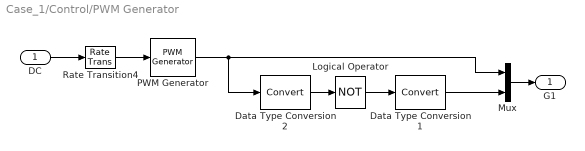
== system Case_1/Control/PWM Generator ==
  DC : Inport
  Data Type Conversion1 : DataTypeConversion  SaturateOnIntegerOverflow=off  RndMeth=Floor
  Data Type Conversion2 : DataTypeConversion  SaturateOnIntegerOverflow=off  RndMeth=Floor
  Logical Operator : Logic  Operator=NOT  AllPortsSameDT=off  OutDataTypeStr=boolean
  Mux : Mux  Inputs=2
  PWM Generator : eePwmGenerator/PWM Generator  CarrCount=Up  Tper=Tsc  Tdelay=0  Ts=Ts
  Rate Transition4 : RateTransition  OutPortSampleTime=Ts
  G1 : Outport  VectorParamsAs1DForOutWhenUnconnected=off
  wires:
  Mux/1 -> G1/1
  Rate Transition4/1 -> PWM Generator/1
  PWM Generator/1 -> Data Type Conversion2/1, Mux/1
  Data Type Conversion1/1 -> Mux/2
  Logical Operator/1 -> Data Type Conversion1/1
  DC/1 -> Rate Transition4/1
  Data Type Conversion2/1 -> Logical Operator/1

== system Case_1/Control/Speed PI Controller ==
  error : Inport
  Constant : Constant  Value=0  SampleTime=Tsc
  Speed controller : eeDiscretePi/Discrete PI Controller with Integral Anti-Windup  Kp=Kpw  Ki=Kiw  x0=0  B=Vdc  A=0  Ts=Tsc
  u : Outport  VectorParamsAs1DForOutWhenUnconnected=off
  wires:
  Constant/1 -> Speed controller/2
  Speed controller/1 -> u/1
  error/1 -> Speed controller/1

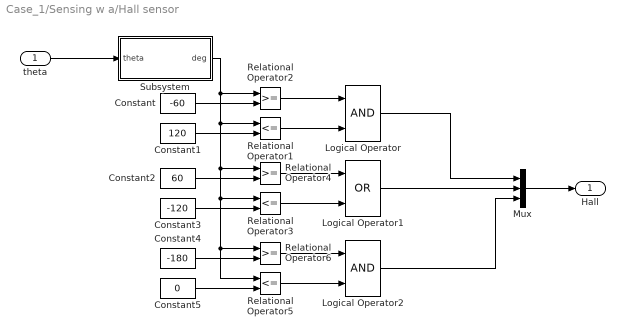
== system Case_1/Sensing w a/Hall sensor ==
  theta : Inport
  Constant : Constant  Value=-60
  Constant1 : Constant  Value=120
  Constant2 : Constant  Value=60
  Constant3 : Constant  Value=-120
  Constant4 : Constant  Value=-180
  Constant5 : Constant  Value=0
  Logical Operator : Logic  AllPortsSameDT=off  OutDataTypeStr=boolean
  Logical Operator1 : Logic  Operator=OR  AllPortsSameDT=off  OutDataTypeStr=boolean
  Logical Operator2 : Logic  AllPortsSameDT=off  OutDataTypeStr=boolean
  Mux : Mux  Inputs=3
  Relational Operator1 : RelationalOperator  Operator=<=
  Relational Operator2 : RelationalOperator
  Relational Operator3 : RelationalOperator  Operator=<=
  Relational Operator4 : RelationalOperator
  Relational Operator5 : RelationalOperator  Operator=<=
  Relational Operator6 : RelationalOperator
  Subsystem : Subsystem
  Hall : Outport  VectorParamsAs1DForOutWhenUnconnected=off
  wires:
  Constant3/1 -> Relational Operator3/2
  Logical Operator2/1 -> Mux/3
  Logical Operator1/1 -> Mux/2
  Logical Operator/1 -> Mux/1
  Relational Operator5/1 -> Logical Operator2/2
  Relational Operator6/1 -> Logical Operator2/1
  Constant4/1 -> Relational Operator6/2
  Constant5/1 -> Relational Operator5/2
  Relational Operator3/1 -> Logical Operator1/2
  Mux/1 -> Hall/1
  Relational Operator2/1 -> Logical Operator/1
  Relational Operator1/1 -> Logical Operator/2
  Subsystem/1(deg) -> Relational Operator4/1, Relational Operator3/1, Relational Operator5/1, Relational Operator6/1, Relational Operator1/1, Relational Operator2/1
  Constant/1 -> Relational Operator2/2
  Relational Operator4/1 -> Logical Operator1/1
  Constant1/1 -> Relational Operator1/2
  Constant2/1 -> Relational Operator4/2
  theta/1 -> Subsystem/1(theta)

== system Case_1/Control/Commutation logic/Bit concatenate ==
  u : Inport
  Gain : Gain  Gain=[4 2 1]  Multiplication=Matrix(K*u)
  Sum of Elements : Sum  Inputs=+
  y : Outport  VectorParamsAs1DForOutWhenUnconnected=off
  wires:
  u/1 -> Gain/1
  Gain/1 -> Sum of Elements/1
  Sum of Elements/1 -> y/1

== system Case_1/Sensing w a/Hall sensor/Subsystem ==
  theta : Inport
  Trigonometric Function : Trigonometry  Operator=sincos
  Trigonometric Function2 : Trigonometry  Operator=atan2
  mech->elec : Gain  Gain=p
  rad->deg : Gain  Gain=180/pi  SaturateOnIntegerOverflow=on  OutDataTypeStr=Inherit: Same as input  ParamDataTypeStr=Inherit: Same as input
  deg : Outport  VectorParamsAs1DForOutWhenUnconnected=off
  wires:
  Trigonometric Function2/1 -> rad->deg/1
  Trigonometric Function/1 -> Trigonometric Function2/1
  theta/1 -> mech->elec/1
  rad->deg/1 -> deg/1
  Trigonometric Function/2 -> Trigonometric Function2/2
  mech->elec/1 -> Trigonometric Function/1
